simulink library "ChimeSignalGeneratorLibBtc"  (R2022b)
settings: Solver=VariableStepAuto  StartTime=0.0  StopTime=10.0  RelTol=1e-3
libraries: simulink x12, dspmathops x3, FeaturePath x1, HandyTextFile x1, RTC x1
(part 1 of 2)
settings Model: Creator=kl13806  LastModifiedBy=kl13806
settings SolverCC: AlgebraicLoopSolver=TrustRegion
settings DebuggingCC: UnconnectedInputMsg=warning  UnconnectedOutputMsg=warning  UnconnectedLineMsg=warning  SFMachineParentedDataDiag=warning
settings ModelReferenceCC: EnableRefExpFcnMdlSchedulingChecks=on
settings RTWCC: DLArmComputeVersion=19.05

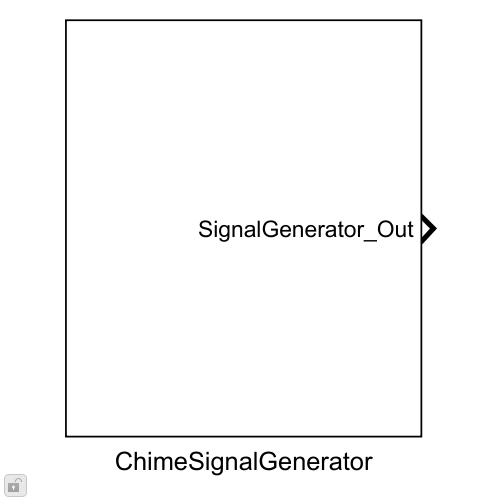
[thumbnail: Simulink's stored preview of the top-level diagram]
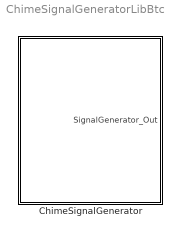
== system ChimeSignalGeneratorLibBtc ==
  ChimeSignalGenerator : Subsystem  mask(Chimes ChimeSignalGenerator){Config=[], FeatureName=SignalGenerator}
      mask prompts: Config "ChimeSignalGeneratorConfig"; FeatureName "Feature path name:"
      mask init:
      | blkh=gcbh;
      | Config=BTConfig.Assert(blkh,Config);
      | 
      | Config.Validate();
      | 
      | BTConfig.InitSetFeatureIfPresent(blkh,'FeatureName');
      | 
      | % Flatten for MFBs
      | frameSize_samples = Config.FrameSizeSamples;
      mask Callback Config: BTConfig.CallbackHideIfPresent(gcbh,{'FeatureName'});
      mask TypeOptions FeatureName: FeaturePath/FeatureName

== system ChimeSignalGeneratorLibBtc/ChimeSignalGenerator ==
  FeaturePath : FeaturePath/FeaturePath  FeatureName=SignalGenerator  IsGroup=off  GroupNumber=-1  IsModule=off  TriggerInit=[345 -266 495 -144]
  For Each Subsystem : Subsystem  TreatAsAtomicUnit=on
  HandyDefaultConfigFile : HandyTextFile/HandyTextFile  TemplateSource=Config  FileSuffix=Init  OpenDialogOnLoad=off  UseThisBlockName=off  TheDefaultText=|  ShowInLibBrowser=on
      | % $(FILENAME) Setup model parameters for each "Init" callback (e.g. update diagram)
      | sample_rate_in_hertz = 44100;
      | frame_size = 32;
      | sysin_channel_count = 2;
  RTC : RTC/RTC  Description=It is LinearSignal generator block  REQ_Priority=RTC_Mask.NormalPriority  RequestAtInit=off  EnableRequest=off  REQElemName1=ChimesMode  REQElemType1=int32  REQElemWidth1=length(Config.SelectMode)  REQElemInitial1=[Config.SelectMode]  REQElemName2=StartingFrequency  REQElemType2=single  REQElemWidth2=length(Config.StartFreqHz)  REQElemInitial2=[Config.StartFreqHz]  REQElemName3=EndingFrequency  REQElemType3=single  REQElemWidth3=length(Config.EndFreqHz)  REQElemInitial3=[Config.EndFreqHz]  REQElemName4=Steps  REQElemType4=single  REQElemWidth4=length(Config.SweepTimeSec)  REQElemInitial4=[Config.SweepTimeSec]  REQElemName5=StartingPhase  REQElemType5=single  REQElemWidth5=length(Config.StartPhaseRad)  REQElemInitial5=[Config.StartPhaseRad]  REQElemName6=ToneGains  REQElemType6=single  REQElemWidth6=length(Config.ToneGains)  REQElemInitial6=[Config.ToneGains]  REQElemName7=RandomNoise  REQElemType7=single  REQElemWidth7=length(Config.RandomNoise)  REQElemInitial7=[Config.RandomNoise]  REQElemName8=CyclesPerSteps  REQElemType8=int32  REQElemWidth8=length(Config.CyclesPerStep)  REQElemInitial8=[Config.CyclesPerStep]  REQElemType9=uint32  REQElemWidth9=1  REQElemInitial9=[]  REQElemType10=uint32  REQElemWidth10=1  REQElemInitial10=[]  EnableResponse=on  EnableRSP_StatusIn=off  RSPElemType1=uint32  RSPElemWidth1=1  RSPElemType2=uint32  RSPElemWidth2=1  RSPElemType3=uint32  RSPElemWidth3=1  RSPElemType4=uint32  RSPElemWidth4=1  RSPElemType5=uint32  RSPElemWidth5=1  RSPElemType6=uint32  RSPElemWidth6=1  RSPElemType7=uint32  RSPElemWidth7=1  RSPElemType8=uint32  RSPElemWidth8=1  RSPElemType9=uint32  RSPElemWidth9=1  RSPElemType10=uint32  RSPElemWidth10=1  EnableNotification=off  EnableNTF_PrepTrig=off  NTFElemType1=uint32  NTFElemWidth1=1  NTFElemType2=uint32  NTFElemWidth2=1  NTFElemType3=uint32  NTFElemWidth3=1  NTFElemType4=uint32  NTFElemWidth4=1  NTFElemType5=uint32  NTFElemWidth5=1  NTFElemType6=uint32  NTFElemWidth6=1  NTFElemType7=uint32  NTFElemWidth7=1  NTFElemType8=uint32  NTFElemWidth8=1  NTFElemType9=uint32  NTFElemWidth9=1  NTFElemType10=uint32  NTFElemWidth10=1  MaskMessageName=Set
  Transpose{,1..7} (8 alike) : Math  Operator=transpose  SignedPower=on
  SignalGenerator_Out : Outport  PortDimensions=[Config.FrameSizeSamples length(Config.SelectMode)]  VectorParamsAs1DForOutWhenUnconnected=off
  wires:
  Transpose7/1 -> For Each Subsystem/7(RandomNoise)  "tone_gains"
  RTC/4 -> Transpose3/1  "steps"
  Transpose6/1 -> For Each Subsystem/8(CyclesPerSteps)  "cycels_per_steps"
  RTC/8 -> Transpose6/1  "cycels_per_steps"
  Transpose5/1 -> For Each Subsystem/2(StartFrequency)  "start_freq"
  Transpose4/1 -> For Each Subsystem/3(EndFrequency)  "end_freq"
  Transpose3/1 -> For Each Subsystem/4(Steps)  "steps"
  Transpose1/1 -> For Each Subsystem/5(StartingPhase)  "start_phase"
  Transpose2/1 -> For Each Subsystem/6(ToneGains)  "tone_gains"
  RTC/7 -> Transpose7/1  "random_noise"
  Transpose/1 -> For Each Subsystem/1(mode)  "chime_mode"
  RTC/1 -> Transpose/1  "chime_mode"
  RTC/6 -> Transpose2/1  "tone_gains"
  RTC/5 -> Transpose1/1  "start_phase"
  RTC/3 -> Transpose4/1  "end_freq"
  RTC/2 -> Transpose5/1  "start_freq"
  For Each Subsystem/1(Out) -> SignalGenerator_Out/1

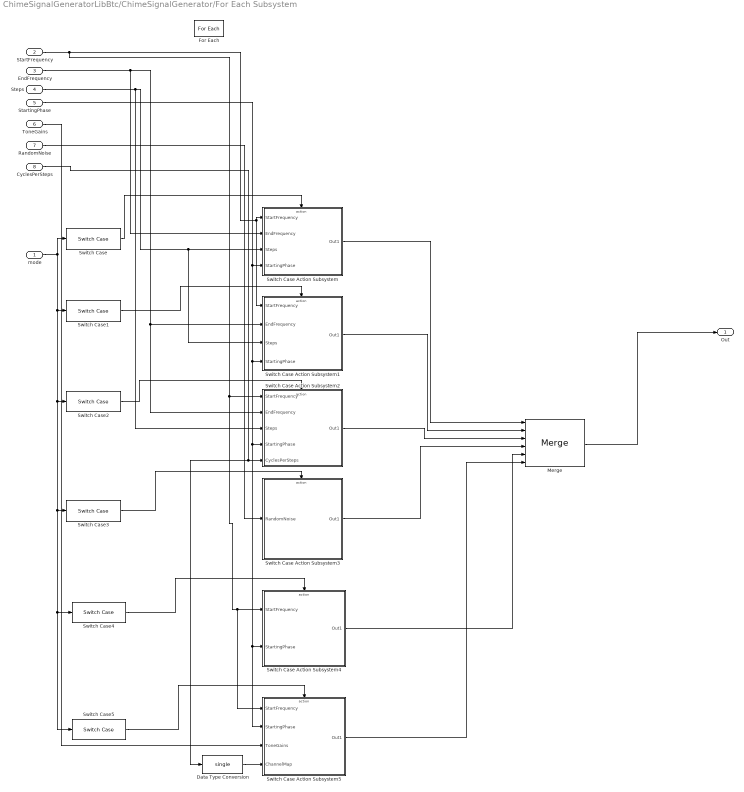
== system ChimeSignalGeneratorLibBtc/ChimeSignalGenerator/For Each Subsystem ==
  mode : Inport  Partition=on  PartitionDimension=2  PartitionWidth=1  PartitionOffset=0
  StartFrequency : Inport  Port=2  Partition=on  PartitionDimension=2  PartitionWidth=2  PartitionOffset=0
  EndFrequency : Inport  Port=3  Partition=on  PartitionDimension=2  PartitionWidth=2  PartitionOffset=0
  Steps : Inport  Port=4  Partition=on  PartitionDimension=2  PartitionWidth=2  PartitionOffset=0
  StartingPhase : Inport  Port=5  Partition=on  PartitionDimension=2  PartitionWidth=2  PartitionOffset=0
  ToneGains : Inport  Port=6  Partition=on  PartitionDimension=2  PartitionWidth=2  PartitionOffset=0
  RandomNoise : Inport  Port=7  Partition=on  PartitionDimension=2  PartitionWidth=2  PartitionOffset=0
  CyclesPerSteps : Inport  Port=8  Partition=on  PartitionDimension=2  PartitionWidth=2  PartitionOffset=0
  Data Type Conversion : DataTypeConversion  OutDataTypeStr=single  SaturateOnIntegerOverflow=off  RndMeth=Floor
  For Each : ForEach  DisableCoverage=on
  Merge : Merge  Inputs=6
  Switch Case : SwitchCase  ShowDefaultCase=off
  Switch Case Action Subsystem : Subsystem  TreatAsAtomicUnit=on
  Switch Case Action Subsystem1 : Subsystem  TreatAsAtomicUnit=on
  Switch Case Action Subsystem2 : Subsystem  TreatAsAtomicUnit=on
  Switch Case Action Subsystem3 : Subsystem  TreatAsAtomicUnit=on
  Switch Case Action Subsystem4 : Subsystem  TreatAsAtomicUnit=on
  Switch Case Action Subsystem5 : Subsystem  TreatAsAtomicUnit=on
  Switch Case1 : SwitchCase  CaseConditions={2}  ShowDefaultCase=off
  Switch Case2 : SwitchCase  CaseConditions={3}  ShowDefaultCase=off
  Switch Case3 : SwitchCase  CaseConditions={4}  ShowDefaultCase=off
  Switch Case4 : SwitchCase  CaseConditions={5}  ShowDefaultCase=off
  Switch Case5 : SwitchCase  CaseConditions={6}  ShowDefaultCase=off
  Out : Outport  ConcatenationDimension=2
  wires:
  StartFrequency/1 -> Switch Case Action Subsystem5/1(StartFrequency), Switch Case Action Subsystem4/1(StartFrequency), Switch Case Action Subsystem2/1(StartFrequency), Switch Case Action Subsystem1/1(StartFrequency), Switch Case Action Subsystem/1(StartFrequency)
  mode/1 -> Switch Case5/1, Switch Case4/1, Switch Case3/1, Switch Case2/1, Switch Case1/1, Switch Case/1
  Switch Case/1 -> Switch Case Action Subsystem/Action
  Switch Case1/1 -> Switch Case Action Subsystem1/Action
  Switch Case2/1 -> Switch Case Action Subsystem2/Action
  Switch Case3/1 -> Switch Case Action Subsystem3/Action
  Switch Case4/1 -> Switch Case Action Subsystem4/Action
  Switch Case5/1 -> Switch Case Action Subsystem5/Action
  Switch Case Action Subsystem3/1(Out1) -> Merge/4
  Switch Case Action Subsystem4/1(Out1) -> Merge/5
  EndFrequency/1 -> Switch Case Action Subsystem/2(EndFrequency), Switch Case Action Subsystem2/2(EndFrequency), Switch Case Action Subsystem1/2(EndFrequency)
  Steps/1 -> Switch Case Action Subsystem1/3(Steps), Switch Case Action Subsystem/3(Steps), Switch Case Action Subsystem2/3(Steps)
  StartingPhase/1 -> Switch Case Action Subsystem/4(StartingPhase), Switch Case Action Subsystem5/2(StartingPhase), Switch Case Action Subsystem4/2(StartingPhase), Switch Case Action Subsystem2/4(StartingPhase), Switch Case Action Subsystem1/4(StartingPhase)
  ToneGains/1 -> Switch Case Action Subsystem5/3(ToneGains)
  RandomNoise/1 -> Switch Case Action Subsystem3/1(RandomNoise)
  CyclesPerSteps/1 -> Data Type Conversion/1, Switch Case Action Subsystem2/5(CyclesPerSteps)
  Switch Case Action Subsystem/1(Out1) -> Merge/1
  Switch Case Action Subsystem1/1(Out1) -> Merge/2
  Switch Case Action Subsystem2/1(Out1) -> Merge/3
  Merge/1 -> Out/1
  Data Type Conversion/1 -> Switch Case Action Subsystem5/4(ChannelMap)
  Switch Case Action Subsystem5/1(Out1) -> Merge/6

== system ChimeSignalGeneratorLibBtc/ChimeSignalGenerator/For Each Subsystem/Switch Case Action Subsystem ==
  StartFrequency : Inport
  EndFrequency : Inport  Port=2
  Steps : Inport  Port=3
  StartingPhase : Inport  Port=4
  Action Port : ActionPort
  Log Sweep Signal Generator : Subsystem
  Out1 : Outport
  wires:
  StartFrequency/1 -> Log Sweep Signal Generator/1(start_freq_Hz)
  EndFrequency/1 -> Log Sweep Signal Generator/2(end_freq_Hz)
  Steps/1 -> Log Sweep Signal Generator/3(sweep_time_sec)
  StartingPhase/1 -> Log Sweep Signal Generator/4(start_phase_rad)
  Log Sweep Signal Generator/1(Log_Sweep_Out) -> Out1/1

== system ChimeSignalGeneratorLibBtc/ChimeSignalGenerator/For Each Subsystem/Switch Case Action Subsystem1 ==
  StartFrequency : Inport
  EndFrequency : Inport  Port=2
  Steps : Inport  Port=3
  StartingPhase : Inport  Port=4
  Action Port : ActionPort
  Linear Sweep Signal Generator : Subsystem
  Out1 : Outport
  wires:
  StartFrequency/1 -> Linear Sweep Signal Generator/1(start_freq_Hz)
  EndFrequency/1 -> Linear Sweep Signal Generator/2(end_freq_Hz)
  Steps/1 -> Linear Sweep Signal Generator/3(sweep_time_sec)
  StartingPhase/1 -> Linear Sweep Signal Generator/4(start_phase_rad)
  Linear Sweep Signal Generator/1(Linear_Sweep_Out) -> Out1/1

== system ChimeSignalGeneratorLibBtc/ChimeSignalGenerator/For Each Subsystem/Switch Case Action Subsystem2 ==
  StartFrequency : Inport
  EndFrequency : Inport  Port=2
  Steps : Inport  Port=3
  StartingPhase : Inport  Port=4
  CyclesPerSteps : Inport  Port=5
  Action Port : ActionPort
  Old Sweep Signal Generator : Subsystem
  Out1 : Outport
  wires:
  StartFrequency/1 -> Old Sweep Signal Generator/1(start_freq_Hz)
  EndFrequency/1 -> Old Sweep Signal Generator/2(end_freq_Hz)
  Steps/1 -> Old Sweep Signal Generator/3(steps)
  StartingPhase/1 -> Old Sweep Signal Generator/4(start_phase_rad)
  CyclesPerSteps/1 -> Old Sweep Signal Generator/5(cycles_per_step)
  Old Sweep Signal Generator/1(Old_sweep_Out) -> Out1/1

== system ChimeSignalGeneratorLibBtc/ChimeSignalGenerator/For Each Subsystem/Switch Case Action Subsystem3 ==
  RandomNoise : Inport
  Action Port : ActionPort
  SigGen_Noise : Subsystem  TreatAsAtomicUnit=on
  Out1 : Outport
  wires:
  RandomNoise/1 -> SigGen_Noise/1(random_noise_input)
  SigGen_Noise/1(Noise_Out) -> Out1/1

== system ChimeSignalGeneratorLibBtc/ChimeSignalGenerator/For Each Subsystem/Switch Case Action Subsystem4 ==
  StartFrequency : Inport
  StartingPhase : Inport  Port=2
  Action Port : ActionPort
  SigGen_Sawtooth : Subsystem  TreatAsAtomicUnit=on
  Out1 : Outport
  wires:
  StartFrequency/1 -> SigGen_Sawtooth/1(StartFreq)
  StartingPhase/1 -> SigGen_Sawtooth/2(start_phase)
  SigGen_Sawtooth/1(Output) -> Out1/1

== system ChimeSignalGeneratorLibBtc/ChimeSignalGenerator/For Each Subsystem/Switch Case Action Subsystem5 ==
  StartFrequency : Inport
  StartingPhase : Inport  Port=2
  ToneGains : Inport  Port=3
  ChannelMap : Inport  Port=4
  Action Port : ActionPort
  SigGen_Multitone : Subsystem
  Out1 : Outport
  wires:
  StartFrequency/1 -> SigGen_Multitone/1(start_freq_Hz)
  SigGen_Multitone/1(Multitone_Out) -> Out1/1  "multitone_output"
  StartingPhase/1 -> SigGen_Multitone/2(start_phase_rad)
  ChannelMap/1 -> SigGen_Multitone/4(ChannelMap)
  ToneGains/1 -> SigGen_Multitone/3(ToneGains)

== system ChimeSignalGeneratorLibBtc/ChimeSignalGenerator/For Each Subsystem/Switch Case Action Subsystem/Log Sweep Signal Generator ==
  start_freq_Hz : Inport
  end_freq_Hz : Inport  Port=2
  sweep_time_sec : Inport  Port=3
  start_phase_rad : Inport  Port=4
  Log Sweep Engine : Subsystem  TreatAsAtomicUnit=on
  Log sweep analysis : Subsystem  Commented=on
  To Workspace : ToWorkspace  Commented=on  VariableName=LogSweepOutput  SampleTime=-1
      settings: Save2DSignal=2-D array (concatenate along first dimension)
  Log_Sweep_Out : Outport  VectorParamsAs1DForOutWhenUnconnected=off
  wires:
  Log Sweep Engine/1(Log_Sweep_Out) -> Log sweep analysis/1(In1), To Workspace/1, Log_Sweep_Out/1
  start_freq_Hz/1 -> Log Sweep Engine/1(start_freq_In)
  end_freq_Hz/1 -> Log Sweep Engine/2(end_freq_In)
  sweep_time_sec/1 -> Log Sweep Engine/3(sweep_time_In)
  start_phase_rad/1 -> Log Sweep Engine/4(start_phase_In)

== system ChimeSignalGeneratorLibBtc/ChimeSignalGenerator/For Each Subsystem/Switch Case Action Subsystem1/Linear Sweep Signal Generator ==
  start_freq_Hz : Inport
  end_freq_Hz : Inport  Port=2
  sweep_time_sec : Inport  Port=3
  start_phase_rad : Inport  Port=4
  Linear Sweep Engine : Subsystem  TreatAsAtomicUnit=on
  Linear sweep analysis : Subsystem  Commented=on
  To Workspace1 : ToWorkspace  Commented=on  VariableName=LinearSweepOutput  SampleTime=-1
      settings: Save2DSignal=2-D array (concatenate along first dimension)
  Linear_Sweep_Out : Outport  VectorParamsAs1DForOutWhenUnconnected=off
  wires:
  start_freq_Hz/1 -> Linear Sweep Engine/1(start_freq_In)
  end_freq_Hz/1 -> Linear Sweep Engine/2(end_freq_In)
  sweep_time_sec/1 -> Linear Sweep Engine/3(sweep_time_In)
  start_phase_rad/1 -> Linear Sweep Engine/4(start_phase_In)
  Linear Sweep Engine/1(Linear_Sweep_Out) -> To Workspace1/1, Linear_Sweep_Out/1, Linear sweep analysis/1(In1)

== system ChimeSignalGeneratorLibBtc/ChimeSignalGenerator/For Each Subsystem/Switch Case Action Subsystem2/Old Sweep Signal Generator ==
  start_freq_Hz : Inport
  end_freq_Hz : Inport  Port=2
  steps : Inport  Port=3
  start_phase_rad : Inport  Port=4
  cycles_per_step : Inport  Port=5
  Old Sweep Engine : Subsystem  TreatAsAtomicUnit=on
  Old sine sweep analysis : Subsystem  Commented=on
  To Workspace5 : ToWorkspace  Commented=on  VariableName=OldSweepOutput  SampleTime=-1
      settings: Save2DSignal=2-D array (concatenate along first dimension)
  Old_sweep_Out : Outport  VectorParamsAs1DForOutWhenUnconnected=off
  wires:
  Old Sweep Engine/1(Old_Sweep_Out) -> To Workspace5/1, Old_sweep_Out/1, Old sine sweep analysis/1(In1)
  start_freq_Hz/1 -> Old Sweep Engine/1(start_freq_In)
  end_freq_Hz/1 -> Old Sweep Engine/2(end_freq_In)
  steps/1 -> Old Sweep Engine/3(steps_In)
  start_phase_rad/1 -> Old Sweep Engine/4(start_phase_In)
  cycles_per_step/1 -> Old Sweep Engine/5(cycles_per_step)

== system ChimeSignalGeneratorLibBtc/ChimeSignalGenerator/For Each Subsystem/Switch Case Action Subsystem3/SigGen_Noise ==
  random_noise_input : Inport
  For Iterator Subsystem : Subsystem  TreatAsAtomicUnit=on
  Noise_Out : Outport  VectorParamsAs1DForOutWhenUnconnected=off
  wires:
  For Iterator Subsystem/1(Out1) -> Noise_Out/1
  random_noise_input/1 -> For Iterator Subsystem/1(InitSeed)  "random_noise"

== system ChimeSignalGeneratorLibBtc/ChimeSignalGenerator/For Each Subsystem/Switch Case Action Subsystem4/SigGen_Sawtooth ==
  StartFreq : Inport
  start_phase : Inport  Port=2
  Add : Sum
  Data Type Conversion : DataTypeConversion  OutDataTypeStr=double  SaturateOnIntegerOverflow=off  RndMeth=Floor
  Data Type Conversion1 : DataTypeConversion  OutDataTypeStr=single  SaturateOnIntegerOverflow=off  RndMeth=Floor
  Divide1 : Product  Inputs=*/
  For Iterator Subsystem : Subsystem  TreatAsAtomicUnit=on
  Mod : Math  Operator=mod  SignedPower=on
  module_phase : Constant  Value=1.0
  sampling_frequency : Constant  Value=Config.FsHz  OutDataTypeStr=single  SampleTime=Inf
  sawtooth_offset : Constant  Value=0.5  OutDataTypeStr=single
  Output : Outport  VectorParamsAs1DForOutWhenUnconnected=off
  wires:
  Mod/1 -> Data Type Conversion1/1  "initial_phase"
  Add/1 -> For Iterator Subsystem/1(IndexStart)  "index_start"
  Data Type Conversion1/1 -> Add/1
  For Iterator Subsystem/1(Out1) -> Output/1
  StartFreq/1 -> Divide1/1
  module_phase/1 -> Mod/2, For Iterator Subsystem/4(ModulePhase)
  sampling_frequency/1 -> Divide1/2
  sawtooth_offset/1 -> For Iterator Subsystem/2(SawtoothOffset), Add/2
  Divide1/1 -> For Iterator Subsystem/3(IncStart)  "inc_start"
  start_phase/1 -> Data Type Conversion/1
  Data Type Conversion/1 -> Mod/1

== system ChimeSignalGeneratorLibBtc/ChimeSignalGenerator/For Each Subsystem/Switch Case Action Subsystem5/SigGen_Multitone ==
  start_freq_Hz : Inport
  start_phase_rad : Inport  Port=2
  ToneGains : Inport  Port=3
  ChannelMap : Inport  Port=4
  Multitone Engine : Subsystem  TreatAsAtomicUnit=on
  Multitone_Out : Outport  VectorParamsAs1DForOutWhenUnconnected=off
  wires:
  ChannelMap/1 -> Multitone Engine/4(ChannelMap)
  Multitone Engine/1(Multitone_Out) -> Multitone_Out/1
  start_phase_rad/1 -> Multitone Engine/2(start_phase_In)  "start_phase"
  start_freq_Hz/1 -> Multitone Engine/1(start_freq_In)  "start_freq"
  ToneGains/1 -> Multitone Engine/3(ToneGains)

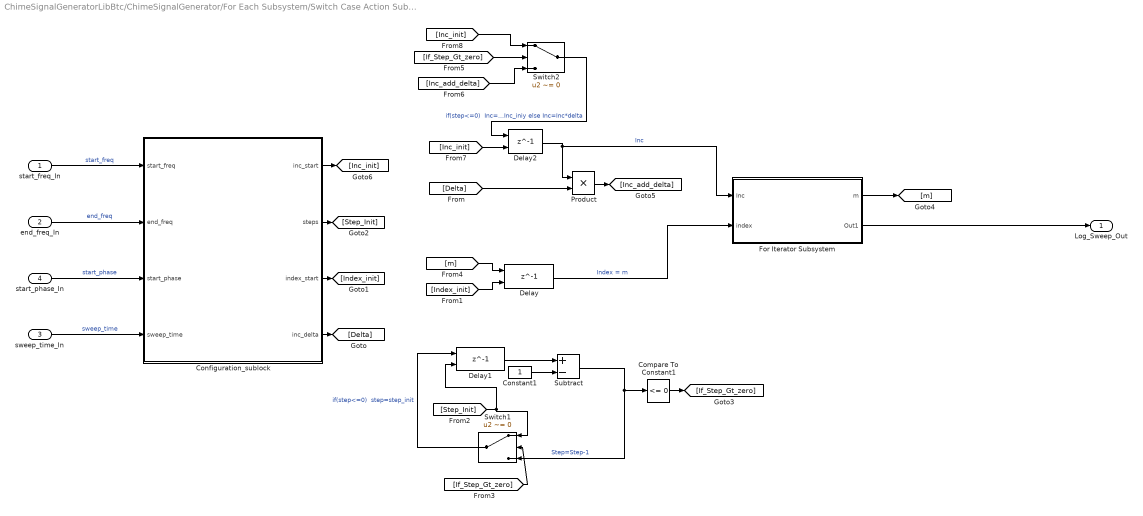
== system ChimeSignalGeneratorLibBtc/ChimeSignalGenerator/For Each Subsystem/Switch Case Action Subsystem/Log Sweep Signal Generator/Log Sweep Engine ==
  start_freq_In : Inport
  end_freq_In : Inport  Port=2
  sweep_time_In : Inport  Port=3
  start_phase_In : Inport  Port=4
  Compare To Constant1 : simulink/Logic and Bit Operations/Compare To Constant  relop=<=  const=0  OutDataTypeStr=boolean
  Configuration_sublock : Subsystem
  Constant1 : Constant  OutDataTypeStr=single
  Delay : Delay  DelayLength=1  InitialConditionSource=Input port
      settings: InputPortMap=u0,p4
  Delay1 : Delay  DelayLength=1  InitialConditionSource=Input port
      settings: InputPortMap=u0,p4
  Delay2 : Delay  DelayLength=1  InitialConditionSource=Input port
      settings: InputPortMap=u0,p4
  For Iterator Subsystem : Subsystem  TreatAsAtomicUnit=on
  Product : Product
  Subtract : Sum  Inputs=+-
  Switch1 : Switch  Criteria=u2 ~= 0  SaturateOnIntegerOverflow=off  InputSameDT=off
  Switch2 : Switch  Criteria=u2 ~= 0  SaturateOnIntegerOverflow=off  InputSameDT=off
  Log_Sweep_Out : Outport  VectorParamsAs1DForOutWhenUnconnected=off
  wires:
  start_freq_In/1 -> Configuration_sublock/1(start_freq)  "start_freq"
  end_freq_In/1 -> Configuration_sublock/2(end_freq)  "end_freq"
  start_phase_In/1 -> Configuration_sublock/3(start_phase)  "start_phase"
  sweep_time_In/1 -> Configuration_sublock/4("sweep_time ")  "sweep_time"
  For Iterator Subsystem/2(Out1) -> Log_Sweep_Out/1
  Configuration_sublock/1(inc_start) -> [Inc_init]
  Configuration_sublock/4(inc_delta) -> [Delta]
  Configuration_sublock/2(steps) -> [Step_Init]
  For Iterator Subsystem/1(m) -> [m]
  Delay/1 -> For Iterator Subsystem/2(index)  "Index = m"
  Subtract/1 -> Switch1/3, Compare To Constant1/1  "Step=Step-1"
  Constant1/1 -> Subtract/2
  Delay1/1 -> Subtract/1
  Switch1/1 -> Delay1/1  "if(step<=0)  step=step_init"
  Delay2/1 -> For Iterator Subsystem/1("Inc "), Product/1  "Inc"
  Configuration_sublock/3(index_start) -> [Index_init]
  [Index_init] -> Delay/2
  [Step_Init] -> Delay1/2, Switch1/1
  Compare To Constant1/1 -> [If_Step_Gt_zero]
  [If_Step_Gt_zero] -> Switch1/2
  [m] -> Delay/1
  [Delta] -> Product/2
  [If_Step_Gt_zero] -> Switch2/2
  Product/1 -> [Inc_add_delta]
  [Inc_add_delta] -> Switch2/3
  [Inc_init] -> Delay2/2
  [Inc_init] -> Switch2/1
  Switch2/1 -> Delay2/1  "if(step<=0)  Inc=Inc_iniy else Inc=Inc*delta"

== system ChimeSignalGeneratorLibBtc/ChimeSignalGenerator/For Each Subsystem/Switch Case Action Subsystem/Log Sweep Signal Generator/Log sweep analysis ==
  In1 : Inport
  Difference : dspmathops/Difference  Run=Yes  dim=Columns  Dimension=1  roundingMode=Floor  overflowMode=off  outputDataTypeStr=Inherit: Same as accumulator  outputMin=[]  outputMax=[]  outputLastDataTypeStr=Inherit: Same as accumulator
  Log Sweep Difference : Scope
  Log Sweep Spectrum Analyzer : SpectrumAnalyzer
  wires:
  Difference/1 -> Log Sweep Difference/1
  In1/1 -> Log Sweep Spectrum Analyzer/1, Difference/1

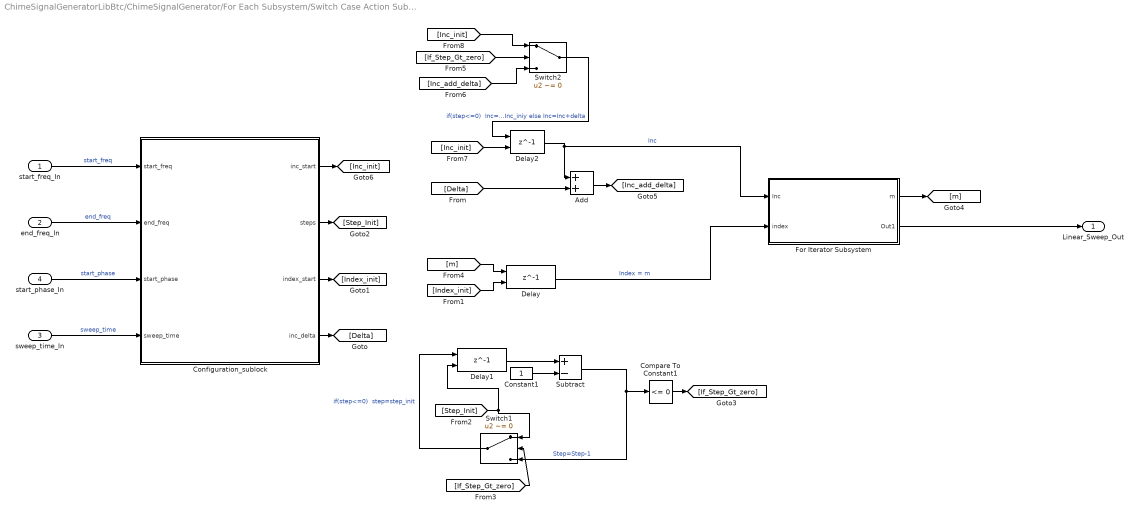
== system ChimeSignalGeneratorLibBtc/ChimeSignalGenerator/For Each Subsystem/Switch Case Action Subsystem1/Linear Sweep Signal Generator/Linear Sweep Engine ==
  start_freq_In : Inport
  end_freq_In : Inport  Port=2
  sweep_time_In : Inport  Port=3
  start_phase_In : Inport  Port=4
  Add : Sum
  Compare To Constant1 : simulink/Logic and Bit Operations/Compare To Constant  relop=<=  const=0  OutDataTypeStr=boolean
  Configuration_sublock : Subsystem
  Constant1 : Constant  OutDataTypeStr=single
  Delay : Delay  DelayLength=1  InitialConditionSource=Input port
      settings: InputPortMap=u0,p4
  Delay1 : Delay  DelayLength=1  InitialConditionSource=Input port
      settings: InputPortMap=u0,p4
  Delay2 : Delay  DelayLength=1  InitialConditionSource=Input port
      settings: InputPortMap=u0,p4
  For Iterator Subsystem : Subsystem  TreatAsAtomicUnit=on
  Subtract : Sum  Inputs=+-
  Switch1 : Switch  Criteria=u2 ~= 0  SaturateOnIntegerOverflow=off  InputSameDT=off
  Switch2 : Switch  Criteria=u2 ~= 0  SaturateOnIntegerOverflow=off  InputSameDT=off
  Linear_Sweep_Out : Outport  VectorParamsAs1DForOutWhenUnconnected=off
  wires:
  Delay2/1 -> For Iterator Subsystem/1("Inc "), Add/1  "Inc"
  Configuration_sublock/4(inc_delta) -> [Delta]
  [Delta] -> Add/2
  [m] -> Delay/1
  Switch1/1 -> Delay1/1  "if(step<=0)  step=step_init"
  [Inc_add_delta] -> Switch2/3
  Delay1/1 -> Subtract/1
  [If_Step_Gt_zero] -> Switch2/2
  [Step_Init] -> Delay1/2, Switch1/1
  start_phase_In/1 -> Configuration_sublock/3(start_phase)  "start_phase"
  Compare To Constant1/1 -> [If_Step_Gt_zero]
  Add/1 -> [Inc_add_delta]
  [Inc_init] -> Delay2/2
  Constant1/1 -> Subtract/2
  Configuration_sublock/1(inc_start) -> [Inc_init]
  [Inc_init] -> Switch2/1
  Switch2/1 -> Delay2/1  "if(step<=0)  Inc=Inc_iniy else Inc=Inc+delta"
  [If_Step_Gt_zero] -> Switch1/2
  Subtract/1 -> Switch1/3, Compare To Constant1/1  "Step=Step-1"
  Delay/1 -> For Iterator Subsystem/2(index)  "Index = m"
  start_freq_In/1 -> Configuration_sublock/1(start_freq)  "start_freq"
  For Iterator Subsystem/1(m) -> [m]
  Configuration_sublock/2(steps) -> [Step_Init]
  [Index_init] -> Delay/2
  For Iterator Subsystem/2(Out1) -> Linear_Sweep_Out/1
  end_freq_In/1 -> Configuration_sublock/2(end_freq)  "end_freq"
  sweep_time_In/1 -> Configuration_sublock/4("sweep_time ")  "sweep_time"
  Configuration_sublock/3(index_start) -> [Index_init]

== system ChimeSignalGeneratorLibBtc/ChimeSignalGenerator/For Each Subsystem/Switch Case Action Subsystem1/Linear Sweep Signal Generator/Linear sweep analysis ==
  In1 : Inport
  Difference : dspmathops/Difference  Run=Yes  dim=Columns  Dimension=1  roundingMode=Floor  overflowMode=off  outputDataTypeStr=Inherit: Same as accumulator  outputMin=[]  outputMax=[]  outputLastDataTypeStr=Inherit: Same as accumulator
  Linear Sweep Difference : Scope
  Linear Sweep Spectrum Analyzer : SpectrumAnalyzer
  wires:
  Difference/1 -> Linear Sweep Difference/1
  In1/1 -> Linear Sweep Spectrum Analyzer/1, Difference/1

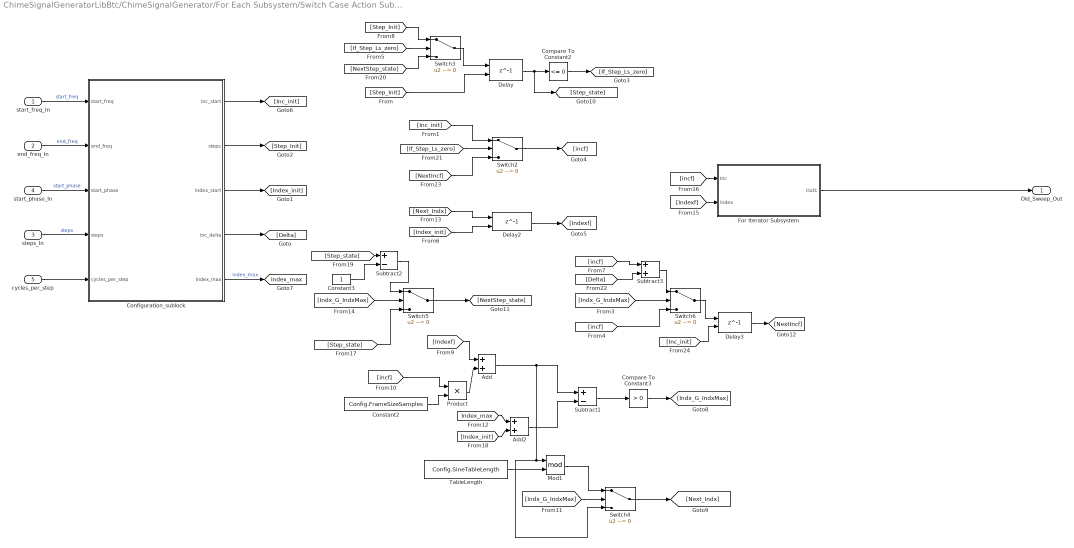
== system ChimeSignalGeneratorLibBtc/ChimeSignalGenerator/For Each Subsystem/Switch Case Action Subsystem2/Old Sweep Signal Generator/Old Sweep Engine ==
  start_freq_In : Inport
  end_freq_In : Inport  Port=2
  steps_In : Inport  Port=3
  start_phase_In : Inport  Port=4
  cycles_per_step : Inport  Port=5
  Add : Sum
  Add2 : Sum  AccumDataTypeStr=single
  Compare To Constant2 : simulink/Logic and Bit Operations/Compare To Constant  relop=<=  const=0  OutDataTypeStr=boolean
  Compare To Constant3 : simulink/Logic and Bit Operations/Compare To Constant  relop=>  const=0  OutDataTypeStr=boolean
  Configuration_sublock : Subsystem
  Constant2 : Constant  Value=Config.FrameSizeSamples  OutDataTypeStr=uint32
  Constant3 : Constant  OutDataTypeStr=single
  Delay : Delay  DelayLength=1  InitialConditionSource=Input port
      settings: InputPortMap=u0,p4
  Delay2 : Delay  DelayLength=1  InitialConditionSource=Input port
      settings: InputPortMap=u0,p4
  Delay3 : Delay  DelayLength=1  InitialConditionSource=Input port
      settings: InputPortMap=u0,p4
  For Iterator Subsystem : Subsystem  TreatAsAtomicUnit=on
  Mod1 : Math  Operator=mod  SignedPower=on
  Product : Product
  Subtract1 : Sum  Inputs=+-
  Subtract2 : Sum  Inputs=+-
  Subtract3 : Sum
  Switch{2..6} (5 alike) : Switch  Criteria=u2 ~= 0  SaturateOnIntegerOverflow=off  InputSameDT=off
  TableLength : Constant  Value=Config.SineTableLength  VectorParams1D=off  OutDataTypeStr=single
  Old_Sweep_Out : Outport  VectorParamsAs1DForOutWhenUnconnected=off
  tag scope: Index_max=global
  wires:
  start_freq_In/1 -> Configuration_sublock/1(start_freq)  "start_freq"
  end_freq_In/1 -> Configuration_sublock/2(end_freq)  "end_freq"
  start_phase_In/1 -> Configuration_sublock/3(start_phase)  "start_phase"
  steps_In/1 -> Configuration_sublock/4("steps ")  "steps"
  For Iterator Subsystem/1(Out1) -> Old_Sweep_Out/1
  Configuration_sublock/1(inc_start) -> [Inc_init]
  Configuration_sublock/4(inc_delta) -> [Delta]
  Configuration_sublock/2(steps) -> [Step_Init]
  Configuration_sublock/3(index_start) -> [Index_init]
  cycles_per_step/1 -> Configuration_sublock/5(cycles_per_step)
  [Indexf] -> For Iterator Subsystem/2(index)
  [incf] -> For Iterator Subsystem/1("Inc ")
  Configuration_sublock/5(index_max) -> [Index_max]  "index_max"
  [Step_Init] -> Delay/2
  Delay/1 -> Compare To Constant2/1, [Step_state]
  Compare To Constant2/1 -> [If_Step_Ls_zero]
  [If_Step_Ls_zero] -> Switch2/2
  [Inc_init] -> Switch2/1
  Switch2/1 -> [incf]
  Delay2/1 -> [Indexf]
  [Index_init] -> Delay2/2
  [If_Step_Ls_zero] -> Switch3/2
  [Step_Init] -> Switch3/1
  Switch3/1 -> Delay/1
  [Indexf] -> Add/1
  [incf] -> Product/1
  Constant2/1 -> Product/2
  Product/1 -> Add/2
  Add/1 -> Switch4/3, Mod1/1, Subtract1/1
  [Index_init] -> Add2/2
  [Index_max] -> Add2/1
  Add2/1 -> Subtract1/2
  Subtract1/1 -> Compare To Constant3/1
  [Indx_G_IndxMax] -> Switch4/2
  TableLength/1 -> Mod1/2
  Mod1/1 -> Switch4/1
  Switch4/1 -> [Next_Indx]
  [Next_Indx] -> Delay2/1
  [Indx_G_IndxMax] -> Switch5/2
  [Step_state] -> Switch5/3
  [Step_state] -> Subtract2/1
  Constant3/1 -> Subtract2/2
  Subtract2/1 -> Switch5/1
  Switch5/1 -> [NextStep_state]
  [NextStep_state] -> Switch3/3
  Compare To Constant3/1 -> [Indx_G_IndxMax]
  [Indx_G_IndxMax] -> Switch6/2
  [incf] -> Switch6/3
  [incf] -> Subtract3/1
  [Delta] -> Subtract3/2
  Subtract3/1 -> Switch6/1
  Switch6/1 -> Delay3/1
  [NextIncf] -> Switch2/3
  [Inc_init] -> Delay3/2
  Delay3/1 -> [NextIncf]

== system ChimeSignalGeneratorLibBtc/ChimeSignalGenerator/For Each Subsystem/Switch Case Action Subsystem2/Old Sweep Signal Generator/Old sine sweep analysis ==
  In1 : Inport
  Difference : dspmathops/Difference  Run=Yes  dim=Columns  Dimension=1  roundingMode=Floor  overflowMode=off  outputDataTypeStr=Inherit: Same as accumulator  outputMin=[]  outputMax=[]  outputLastDataTypeStr=Inherit: Same as accumulator
  Old Sweep Difference : Scope
  Old Sweep Spectrum Analyzer : SpectrumAnalyzer
  wires:
  Difference/1 -> Old Sweep Difference/1
  In1/1 -> Old Sweep Spectrum Analyzer/1, Difference/1

== system ChimeSignalGeneratorLibBtc/ChimeSignalGenerator/For Each Subsystem/Switch Case Action Subsystem3/SigGen_Noise/For Iterator Subsystem ==
  InitSeed : Inport
  Add1 : Sum
  Constant4 : Constant
  Data Type Conversion : DataTypeConversion  OutDataTypeStr=uint32  SaturateOnIntegerOverflow=off  RndMeth=Floor
  Delay1 : Delay  DelayLength=1  InitialConditionSource=Input port
      settings: InputPortMap=u0,p4
  For Iterator : ForIterator  IterationLimit=Config.FrameSizeSamples
  MATLAB Function : MATLAB Function  TreatAsAtomicUnit=on
  Multiply : Product
  Multiply1 : Product
  Subtract : Sum  Inputs=+-
  rnParam1 : Constant  Value=4.656612873077393e-010
  rnParam2 : Constant  Value=1664525
  rnParam3 : Constant  Value=1013904223
  Out1 : Outport  VectorParamsAs1DForOutWhenUnconnected=off
  wires:
  For Iterator/1 -> MATLAB Function/1(Index)
  Data Type Conversion/1 -> Multiply1/1, Multiply/2
  rnParam1/1 -> Multiply/1
  Multiply/1 -> Subtract/1
  rnParam2/1 -> Multiply1/2
  Constant4/1 -> Subtract/2
  Subtract/1 -> MATLAB Function/2(Data)
  Multiply1/1 -> Add1/1
  rnParam3/1 -> Add1/2
  Add1/1 -> Delay1/1
  Delay1/1 -> Data Type Conversion/1
  InitSeed/1 -> Delay1/2
  MATLAB Function/1(y) -> Out1/1

== system ChimeSignalGeneratorLibBtc/ChimeSignalGenerator/For Each Subsystem/Switch Case Action Subsystem4/SigGen_Sawtooth/For Iterator Subsystem ==
  IndexStart : Inport
  SawtoothOffset : Inport  Port=2
  IncStart : Inport  Port=3
  ModulePhase : Inport  Port=4
  Add1 : Sum
  Constant : Constant  Value=-2.0
  Delay : Delay  DelayLength=1  InitialConditionSource=Input port
      settings: InputPortMap=u0,p4
  For Iterator : ForIterator  IterationLimit=Config.FrameSizeSamples
  MATLAB Function : MATLAB Function  TreatAsAtomicUnit=on
  Mod1 : Math  Operator=mod  SignedPower=on
  Multiply : Product
  Subtract : Sum  Inputs=+-
  Out1 : Outport  VectorParamsAs1DForOutWhenUnconnected=off
  wires:
  MATLAB Function/1(y) -> Out1/1
  ModulePhase/1 -> Mod1/2
  SawtoothOffset/1 -> Subtract/2
  IndexStart/1 -> Delay/2  "index_start"
  IncStart/1 -> Add1/2  "inc_start"
  Delay/1 -> Add1/1, Subtract/1  "phase"
  Subtract/1 -> Multiply/1
  Constant/1 -> Multiply/2
  Add1/1 -> Mod1/1
  Mod1/1 -> Delay/1  "initial_phase"
  Multiply/1 -> MATLAB Function/2(Data)
  For Iterator/1 -> MATLAB Function/1(Index)

== system ChimeSignalGeneratorLibBtc/ChimeSignalGenerator/For Each Subsystem/Switch Case Action Subsystem5/SigGen_Multitone/Multitone Engine ==
  start_freq_In : Inport
  start_phase_In : Inport  Port=2
  ToneGains : Inport  Port=3
  ChannelMap : Inport  Port=4
  Add : Sum
  Configuration_sublock : Subsystem
  Delay : Delay  DelayLength=1  InitialConditionSource=Input port
      settings: InputPortMap=u0,p4
  For Iterator Subsystem : Subsystem  TreatAsAtomicUnit=on
  Multitone_Out : Outport  VectorParamsAs1DForOutWhenUnconnected=off
  wires:
  ChannelMap/1 -> For Iterator Subsystem/4(ChannelMap)
  Configuration_sublock/2(index_start) -> [Index_init]  "index_start"
  [Index_init] -> Delay/2
  [m] -> Delay/1
  Delay/1 -> For Iterator Subsystem/2(index)  "m1"
  ToneGains/1 -> For Iterator Subsystem/3(ToneGains)
  [Inc_init] -> Add/1  "inc"
  Add/1 -> For Iterator Subsystem/1("Inc ")
  [Delta] -> Add/2
  For Iterator Subsystem/1(m) -> [m]
  Configuration_sublock/3(inc_delta) -> [Delta]
  Configuration_sublock/1(inc_start) -> [Inc_init]
  For Iterator Subsystem/2(Out1) -> Multitone_Out/1
  start_phase_In/1 -> Configuration_sublock/2(start_phase)  "start_phase"
  start_freq_In/1 -> Configuration_sublock/1(start_freq)  "start_freq"

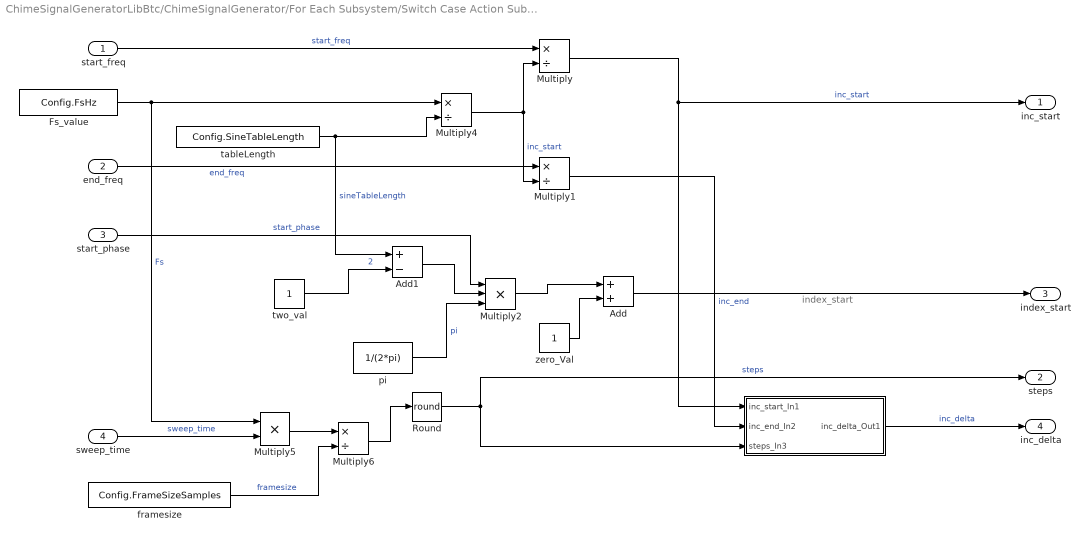
== system ChimeSignalGeneratorLibBtc/ChimeSignalGenerator/For Each Subsystem/Switch Case Action Subsystem/Log Sweep Signal Generator/Log Sweep Engine/Configuration_sublock ==
  note: index_start
  start_freq : Inport
  end_freq : Inport  Port=2
  start_phase : Inport  Port=3
  "sweep_time " : Inport  Port=4
  " " : Subsystem  TreatAsAtomicUnit=on
  Add : Sum
  Add1 : Sum  Inputs=+-
  Fs_value : Constant  Value=Config.FsHz  OutDataTypeStr=single
  Multiply{,1,4,6} (4 alike) : Product  Inputs=*/
  Multiply2 : Product  Inputs=***
  Multiply5 : Product  Inputs=**
  Round : Rounding  Operator=round
  framesize : Constant  Value=Config.FrameSizeSamples  VectorParams1D=off  OutDataTypeStr=uint32
  pi : Constant  Value=1/(2*pi)  VectorParams1D=off  OutDataTypeStr=single
  tableLength : Constant  Value=Config.SineTableLength  VectorParams1D=off  OutDataTypeStr=single
  two_val : Constant  VectorParams1D=off  OutDataTypeStr=uint32
  zero_Val : Constant  VectorParams1D=off  OutDataTypeStr=single
  inc_start : Outport  VectorParamsAs1DForOutWhenUnconnected=off
  steps : Outport  Port=2  VectorParamsAs1DForOutWhenUnconnected=off
  index_start : Outport  Port=3  VectorParamsAs1DForOutWhenUnconnected=off
  inc_delta : Outport  Port=4  VectorParamsAs1DForOutWhenUnconnected=off
  wires:
  start_phase/1 -> Multiply2/1  "start_phase"
  tableLength/1 -> Multiply4/2, Add1/1  "sineTableLength"
  two_val/1 -> Add1/2  "2"
  pi/1 -> Multiply2/3  "pi"
  Add1/1 -> Multiply2/2
  zero_Val/1 -> Add/2
  Fs_value/1 -> Multiply5/1, Multiply4/1  "Fs"
  Multiply2/1 -> Add/1
  start_freq/1 -> Multiply/1  "start_freq"
  end_freq/1 -> Multiply1/1  "end_freq"
  Add/1 -> index_start/1
  Multiply/1 -> " "/1(inc_start_In1), inc_start/1  "inc_start"
  Multiply4/1 -> Multiply1/2, Multiply/2  "inc_start"
  Multiply1/1 -> " "/2(inc_end_In2)  "inc_end"
  "sweep_time "/1 -> Multiply5/2  "sweep_time"
  Multiply5/1 -> Multiply6/1
  framesize/1 -> Multiply6/2  "framesize"
  Multiply6/1 -> Round/1
  Round/1 -> " "/3(steps_In3), steps/1  "steps"
  " "/1(inc_delta_Out1) -> inc_delta/1  "inc_delta"

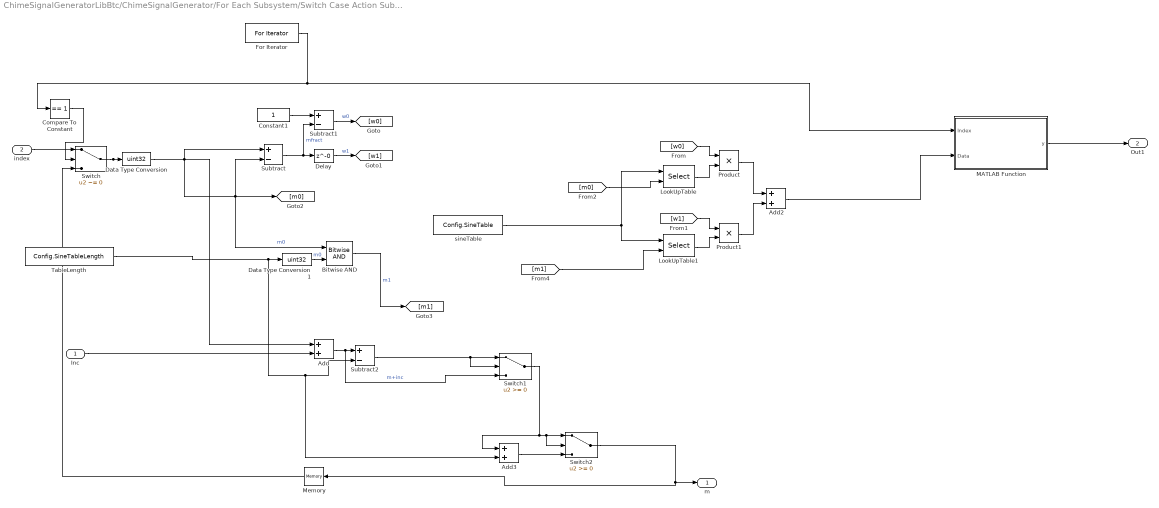
== system ChimeSignalGeneratorLibBtc/ChimeSignalGenerator/For Each Subsystem/Switch Case Action Subsystem/Log Sweep Signal Generator/Log Sweep Engine/For Iterator Subsystem ==
  "Inc " : Inport
  index : Inport  Port=2
  Add : Sum
  Add2 : Sum
  Add3 : Sum
  Bitwise AND : simulink/Logic and Bit Operations/Bitwise Operator  logicop=AND  UseBitMask=off  NumInputPorts=2  BitMask=bin2dec('11011001')  BitMaskRealWorld=Stored Integer
  Compare To Constant : simulink/Logic and Bit Operations/Compare To Constant  relop===  const=1  OutDataTypeStr=boolean
  Constant1 : Constant  OutDataTypeStr=single
  Data Type Conversion : DataTypeConversion  OutDataTypeStr=uint32  SaturateOnIntegerOverflow=off  RndMeth=Floor
  Data Type Conversion1 : DataTypeConversion  OutDataTypeStr=uint32  SaturateOnIntegerOverflow=off  RndMeth=Floor
  Delay : Delay  DelayLength=0
  For Iterator : ForIterator  ResetStates=reset  IterationLimit=Config.FrameSizeSamples
  LookUpTable : Selector  IndexMode=Zero-based  InputPortWidth=Config.SineTableLength  IndexOptions=Index vector (port)  Indices=[1 3]  OutputSizes=1
  LookUpTable1 : Selector  IndexMode=Zero-based  InputPortWidth=Config.SineTableLength  IndexOptions=Index vector (port)  Indices=[1 3]  OutputSizes=1
  MATLAB Function : MATLAB Function  TreatAsAtomicUnit=on
  Memory : Memory  InheritSampleTime=on
  Product : Product
  Product1 : Product
  Subtract : Sum  Inputs=+-  OutDataTypeStr=single
  Subtract1 : Sum  Inputs=+-  OutDataTypeStr=single
  Subtract2 : Sum  Inputs=+-
  Switch : Switch  Criteria=u2 ~= 0  SaturateOnIntegerOverflow=off  InputSameDT=off
  Switch1 : Switch  SaturateOnIntegerOverflow=off  InputSameDT=off
  Switch2 : Switch  SaturateOnIntegerOverflow=off  InputSameDT=off
  TableLength : Constant  Value=Config.SineTableLength  VectorParams1D=off  OutDataTypeStr=single
  sineTable : Constant  Value=Config.SineTable  OutDataTypeStr=single
  m : Outport  VectorParamsAs1DForOutWhenUnconnected=off
  Out1 : Outport  Port=2  VectorParamsAs1DForOutWhenUnconnected=off
  wires:
  Add2/1 -> MATLAB Function/2(Data)
  TableLength/1 -> Data Type Conversion1/1, Add3/2, Subtract2/2
  Compare To Constant/1 -> Switch/2
  index/1 -> Switch/1
  Switch/1 -> Add/1, Data Type Conversion/1
  Add/1 -> Switch1/3, Subtract2/1  "m+inc"
  For Iterator/1 -> MATLAB Function/1(Index), Compare To Constant/1
  Memory/1 -> Switch/3
  Data Type Conversion/1 -> Bitwise AND/1, Subtract/2, [m0], Subtract/1  "m0"
  Subtract/1 -> Delay/1, Subtract1/2  "mfract"
  Constant1/1 -> Subtract1/1
  Subtract1/1 -> [w0]  "w0"
  Delay/1 -> [w1]  "w1"
  sineTable/1 -> LookUpTable1/1, LookUpTable/1
  [m0] -> LookUpTable/2
  [w0] -> Product/1
  LookUpTable/1 -> Product/2
  [m1] -> LookUpTable1/2
  [w1] -> Product1/1
  LookUpTable1/1 -> Product1/2
  Product/1 -> Add2/1
  Product1/1 -> Add2/2
  MATLAB Function/1(y) -> Out1/1
  "Inc "/1 -> Add/2
  Data Type Conversion1/1 -> Bitwise AND/2  "m0"
  Switch1/1 -> Add3/1, Switch2/2, Switch2/1
  Switch2/1 -> Memory/1, m/1
  Subtract2/1 -> Switch1/1, Switch1/2
  Add3/1 -> Switch2/3
  Bitwise AND/1 -> [m1]  "m1"

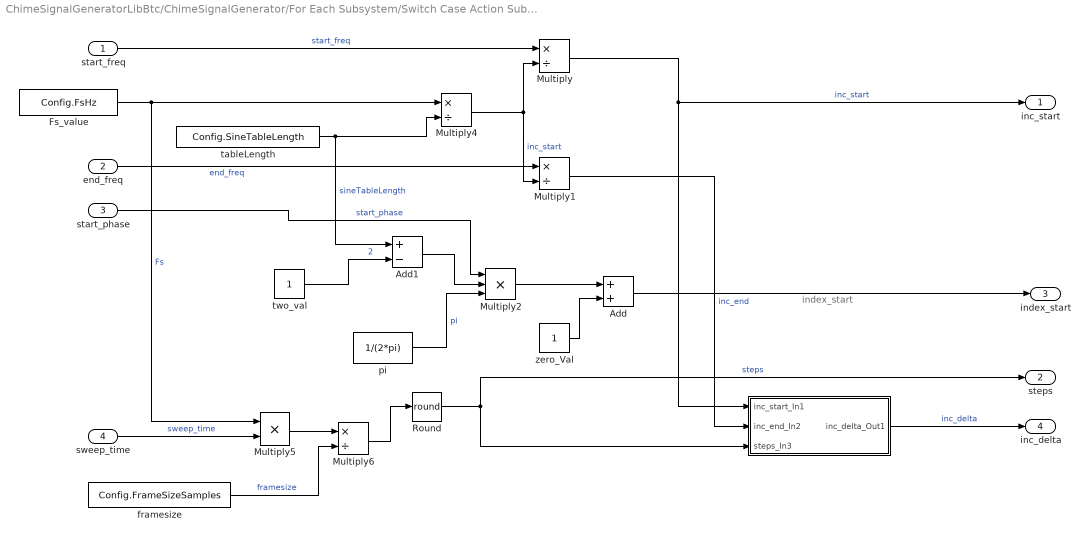
== system ChimeSignalGeneratorLibBtc/ChimeSignalGenerator/For Each Subsystem/Switch Case Action Subsystem1/Linear Sweep Signal Generator/Linear Sweep Engine/Configuration_sublock ==
  note: index_start
  start_freq : Inport
  end_freq : Inport  Port=2
  start_phase : Inport  Port=3
  "sweep_time " : Inport  Port=4
  " " : Subsystem  TreatAsAtomicUnit=on
  Add : Sum
  Add1 : Sum  Inputs=+-
  Fs_value : Constant  Value=Config.FsHz  OutDataTypeStr=single
  Multiply{,1,4,6} (4 alike) : Product  Inputs=*/
  Multiply2 : Product  Inputs=***
  Multiply5 : Product  Inputs=**
  Round : Rounding  Operator=round
  framesize : Constant  Value=Config.FrameSizeSamples  VectorParams1D=off  OutDataTypeStr=uint32
  pi : Constant  Value=1/(2*pi)  VectorParams1D=off  OutDataTypeStr=single
  tableLength : Constant  Value=Config.SineTableLength  VectorParams1D=off  OutDataTypeStr=single
  two_val : Constant  VectorParams1D=off  OutDataTypeStr=uint32
  zero_Val : Constant  VectorParams1D=off  OutDataTypeStr=single
  inc_start : Outport  VectorParamsAs1DForOutWhenUnconnected=off
  steps : Outport  Port=2  VectorParamsAs1DForOutWhenUnconnected=off
  index_start : Outport  Port=3  VectorParamsAs1DForOutWhenUnconnected=off
  inc_delta : Outport  Port=4  VectorParamsAs1DForOutWhenUnconnected=off
  wires:
  Add1/1 -> Multiply2/2
  zero_Val/1 -> Add/2
  two_val/1 -> Add1/2  "2"
  pi/1 -> Multiply2/3  "pi"
  Fs_value/1 -> Multiply5/1, Multiply4/1  "Fs"
  Multiply2/1 -> Add/1
  tableLength/1 -> Multiply4/2, Add1/1  "sineTableLength"
  start_freq/1 -> Multiply/1  "start_freq"
  start_phase/1 -> Multiply2/1  "start_phase"
  end_freq/1 -> Multiply1/1  "end_freq"
  Add/1 -> index_start/1
  Multiply/1 -> " "/1(inc_start_In1), inc_start/1  "inc_start"
  Multiply4/1 -> Multiply1/2, Multiply/2  "inc_start"
  Multiply1/1 -> " "/2(inc_end_In2)  "inc_end"
  "sweep_time "/1 -> Multiply5/2  "sweep_time"
  Multiply5/1 -> Multiply6/1
  framesize/1 -> Multiply6/2  "framesize"
  Multiply6/1 -> Round/1
  Round/1 -> " "/3(steps_In3), steps/1  "steps"
  " "/1(inc_delta_Out1) -> inc_delta/1  "inc_delta"

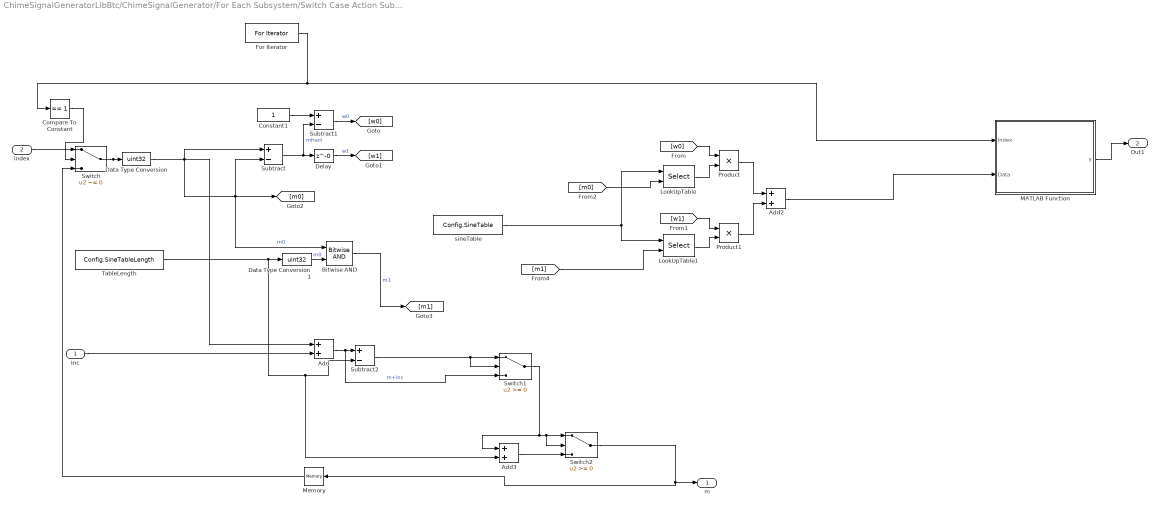
== system ChimeSignalGeneratorLibBtc/ChimeSignalGenerator/For Each Subsystem/Switch Case Action Subsystem1/Linear Sweep Signal Generator/Linear Sweep Engine/For Iterator Subsystem ==
  "Inc " : Inport
  index : Inport  Port=2
  Add : Sum
  Add2 : Sum
  Add3 : Sum
  Bitwise AND : simulink/Logic and Bit Operations/Bitwise Operator  logicop=AND  UseBitMask=off  NumInputPorts=2  BitMask=bin2dec('11011001')  BitMaskRealWorld=Stored Integer
  Compare To Constant : simulink/Logic and Bit Operations/Compare To Constant  relop===  const=1  OutDataTypeStr=boolean
  Constant1 : Constant  OutDataTypeStr=single
  Data Type Conversion : DataTypeConversion  OutDataTypeStr=uint32  SaturateOnIntegerOverflow=off  RndMeth=Floor
  Data Type Conversion1 : DataTypeConversion  OutDataTypeStr=uint32  SaturateOnIntegerOverflow=off  RndMeth=Floor
  Delay : Delay  DelayLength=0
  For Iterator : ForIterator  ResetStates=reset  IterationLimit=Config.FrameSizeSamples
  LookUpTable : Selector  IndexMode=Zero-based  InputPortWidth=Config.SineTableLength  IndexOptions=Index vector (port)  Indices=[1 3]  OutputSizes=1
  LookUpTable1 : Selector  IndexMode=Zero-based  InputPortWidth=Config.SineTableLength  IndexOptions=Index vector (port)  Indices=[1 3]  OutputSizes=1
  MATLAB Function : MATLAB Function  TreatAsAtomicUnit=on
  Memory : Memory  InheritSampleTime=on
  Product : Product
  Product1 : Product
  Subtract : Sum  Inputs=+-  OutDataTypeStr=single
  Subtract1 : Sum  Inputs=+-  OutDataTypeStr=single
  Subtract2 : Sum  Inputs=+-
  Switch : Switch  Criteria=u2 ~= 0  SaturateOnIntegerOverflow=off  InputSameDT=off
  Switch1 : Switch  SaturateOnIntegerOverflow=off  InputSameDT=off
  Switch2 : Switch  SaturateOnIntegerOverflow=off  InputSameDT=off
  TableLength : Constant  Value=Config.SineTableLength  VectorParams1D=off  OutDataTypeStr=single
  sineTable : Constant  Value=Config.SineTable  OutDataTypeStr=single
  m : Outport  VectorParamsAs1DForOutWhenUnconnected=off
  Out1 : Outport  Port=2  VectorParamsAs1DForOutWhenUnconnected=off
  wires:
  Add2/1 -> MATLAB Function/2(Data)
  TableLength/1 -> Data Type Conversion1/1, Add3/2, Subtract2/2
  Compare To Constant/1 -> Switch/2
  index/1 -> Switch/1
  Switch/1 -> Add/1, Data Type Conversion/1
  Add/1 -> Switch1/3, Subtract2/1  "m+inc"
  For Iterator/1 -> MATLAB Function/1(Index), Compare To Constant/1
  Memory/1 -> Switch/3
  Data Type Conversion/1 -> Bitwise AND/1, Subtract/2, [m0], Subtract/1  "m0"
  Subtract/1 -> Delay/1, Subtract1/2  "mfract"
  Constant1/1 -> Subtract1/1
  Subtract1/1 -> [w0]  "w0"
  Delay/1 -> [w1]  "w1"
  sineTable/1 -> LookUpTable1/1, LookUpTable/1
  [m0] -> LookUpTable/2
  [w0] -> Product/1
  LookUpTable/1 -> Product/2
  [m1] -> LookUpTable1/2
  [w1] -> Product1/1
  LookUpTable1/1 -> Product1/2
  Product/1 -> Add2/1
  Product1/1 -> Add2/2
  MATLAB Function/1(y) -> Out1/1
  "Inc "/1 -> Add/2
  Data Type Conversion1/1 -> Bitwise AND/2  "m0"
  Switch1/1 -> Add3/1, Switch2/2, Switch2/1
  Switch2/1 -> Memory/1, m/1
  Subtract2/1 -> Switch1/1, Switch1/2
  Add3/1 -> Switch2/3
  Bitwise AND/1 -> [m1]  "m1"

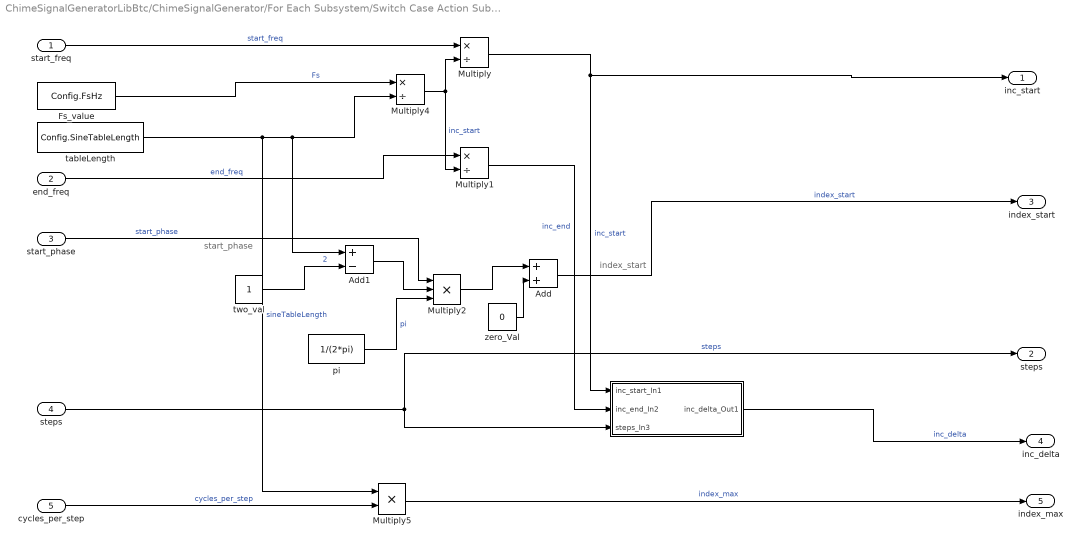
== system ChimeSignalGeneratorLibBtc/ChimeSignalGenerator/For Each Subsystem/Switch Case Action Subsystem2/Old Sweep Signal Generator/Old Sweep Engine/Configuration_sublock ==
  note: index_start
  note: start_phase
  start_freq : Inport
  end_freq : Inport  Port=2
  start_phase : Inport  Port=3
  "steps " : Inport  Port=4
  cycles_per_step : Inport  Port=5
  " " : Subsystem  TreatAsAtomicUnit=on
  Add : Sum
  Add1 : Sum  Inputs=+-
  Fs_value : Constant  Value=Config.FsHz  OutDataTypeStr=single
  Multiply : Product  Inputs=*/
  Multiply1 : Product  Inputs=*/
  Multiply2 : Product  Inputs=***
  Multiply4 : Product  Inputs=*/
  Multiply5 : Product  Inputs=**
  pi : Constant  Value=1/(2*pi)  VectorParams1D=off  OutDataTypeStr=single
  tableLength : Constant  Value=Config.SineTableLength  OutDataTypeStr=single
  two_val : Constant  VectorParams1D=off  OutDataTypeStr=uint32
  zero_Val : Constant  Value=0  OutDataTypeStr=uint32
  inc_start : Outport  VectorParamsAs1DForOutWhenUnconnected=off
  steps : Outport  Port=2  VectorParamsAs1DForOutWhenUnconnected=off
  index_start : Outport  Port=3  VectorParamsAs1DForOutWhenUnconnected=off
  inc_delta : Outport  Port=4  VectorParamsAs1DForOutWhenUnconnected=off
  index_max : Outport  Port=5  VectorParamsAs1DForOutWhenUnconnected=off
  wires:
  start_phase/1 -> Multiply2/1  "start_phase"
  tableLength/1 -> Multiply5/1, Multiply4/2, Add1/1  "sineTableLength"
  two_val/1 -> Add1/2  "2"
  pi/1 -> Multiply2/3  "pi"
  Add1/1 -> Multiply2/2
  Add/1 -> index_start/1  "index_start"
  cycles_per_step/1 -> Multiply5/2  "cycles_per_step"
  Multiply5/1 -> index_max/1  "index_max"
  " "/1(inc_delta_Out1) -> inc_delta/1  "inc_delta"
  "steps "/1 -> " "/3(steps_In3), steps/1  "steps"
  Multiply1/1 -> " "/2(inc_end_In2)  "inc_end"
  Multiply4/1 -> Multiply/2, Multiply1/2  "inc_start"
  Multiply/1 -> inc_start/1, " "/1(inc_start_In1)  "inc_start"
  end_freq/1 -> Multiply1/1  "end_freq"
  start_freq/1 -> Multiply/1  "start_freq"
  Multiply2/1 -> Add/1
  Fs_value/1 -> Multiply4/1  "Fs"
  zero_Val/1 -> Add/2

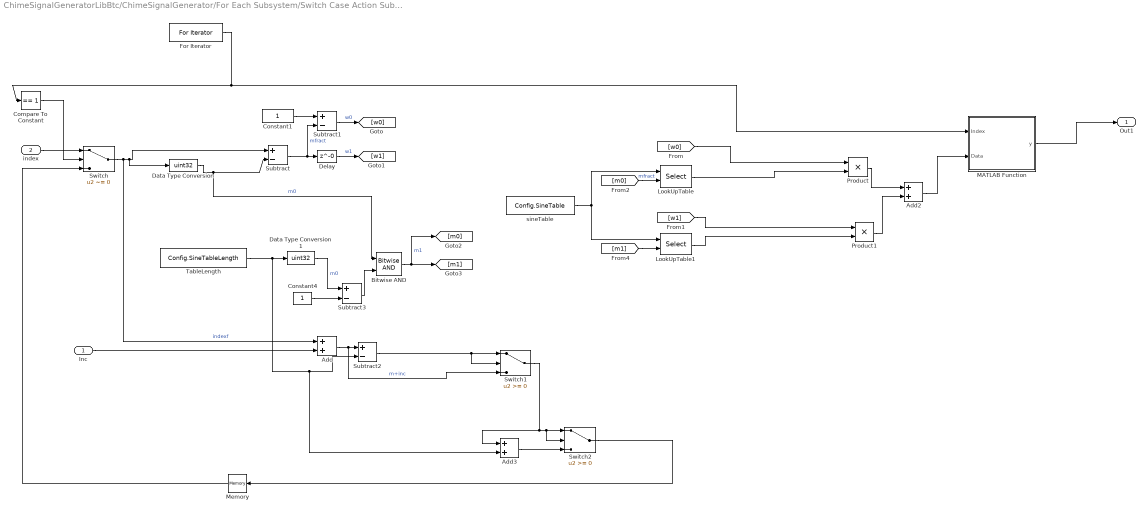
== system ChimeSignalGeneratorLibBtc/ChimeSignalGenerator/For Each Subsystem/Switch Case Action Subsystem2/Old Sweep Signal Generator/Old Sweep Engine/For Iterator Subsystem ==
  "Inc " : Inport
  index : Inport  Port=2
  Add : Sum
  Add2 : Sum
  Add3 : Sum
  Bitwise AND : simulink/Logic and Bit Operations/Bitwise Operator  logicop=AND  UseBitMask=off  NumInputPorts=2  BitMask=bin2dec('11011001')  BitMaskRealWorld=Stored Integer
  Compare To Constant : simulink/Logic and Bit Operations/Compare To Constant  relop===  const=1  OutDataTypeStr=boolean
  Constant1 : Constant  OutDataTypeStr=single
  Constant4 : Constant  OutDataTypeStr=uint32
  Data Type Conversion : DataTypeConversion  OutDataTypeStr=uint32  SaturateOnIntegerOverflow=off  RndMeth=Floor
  Data Type Conversion1 : DataTypeConversion  OutDataTypeStr=uint32  SaturateOnIntegerOverflow=off  RndMeth=Floor
  Delay : Delay  DelayLength=0
  For Iterator : ForIterator  ResetStates=reset  IterationLimit=Config.FrameSizeSamples
  LookUpTable : Selector  IndexMode=Zero-based  InputPortWidth=Config.SineTableLength  IndexOptions=Index vector (port)  Indices=[1 3]  OutputSizes=1
  LookUpTable1 : Selector  IndexMode=Zero-based  InputPortWidth=Config.SineTableLength  IndexOptions=Index vector (port)  Indices=[1 3]  OutputSizes=1
  MATLAB Function : MATLAB Function  TreatAsAtomicUnit=on
  Memory : Memory  InheritSampleTime=on
  Product : Product
  Product1 : Product
  Subtract : Sum  Inputs=+-  OutDataTypeStr=single
  Subtract1 : Sum  Inputs=+-  OutDataTypeStr=single
  Subtract2 : Sum  Inputs=+-
  Subtract3 : Sum  Inputs=+-
  Switch : Switch  Criteria=u2 ~= 0  SaturateOnIntegerOverflow=off  InputSameDT=off
  Switch1 : Switch  SaturateOnIntegerOverflow=off  InputSameDT=off
  Switch2 : Switch  SaturateOnIntegerOverflow=off  InputSameDT=off
  TableLength : Constant  Value=Config.SineTableLength  VectorParams1D=off  OutDataTypeStr=single
  sineTable : Constant  Value=Config.SineTable  OutDataTypeStr=single
  Out1 : Outport  VectorParamsAs1DForOutWhenUnconnected=off
  wires:
  Bitwise AND/1 -> [m0], [m1]  "m1"
  Add3/1 -> Switch2/3
  Subtract2/1 -> Switch1/2, Switch1/1
  Switch2/1 -> Memory/1
  Switch1/1 -> Switch2/1, Switch2/2, Add3/1
  "Inc "/1 -> Add/2
  MATLAB Function/1(y) -> Out1/1
  Product1/1 -> Add2/2
  Product/1 -> Add2/1
  LookUpTable1/1 -> Product1/2
  [w1] -> Product1/1
  [m1] -> LookUpTable1/2
  LookUpTable/1 -> Product/2
  [w0] -> Product/1
  sineTable/1 -> LookUpTable1/1, LookUpTable/1
  Delay/1 -> [w1]  "w1"
  Subtract1/1 -> [w0]  "w0"
  Constant1/1 -> Subtract1/1
  Subtract/1 -> Subtract1/2, Delay/1  "mfract"
  Data Type Conversion/1 -> Subtract/2, Bitwise AND/1  "m0"
  Memory/1 -> Switch/3
  For Iterator/1 -> MATLAB Function/1(Index), Compare To Constant/1
  Add/1 -> Subtract2/1, Switch1/3  "m+inc"
  Switch/1 -> Data Type Conversion/1, Subtract/1, Add/1  "indexf"
  index/1 -> Switch/1
  Compare To Constant/1 -> Switch/2
  TableLength/1 -> Subtract2/2, Add3/2, Data Type Conversion1/1
  Add2/1 -> MATLAB Function/2(Data)
  Data Type Conversion1/1 -> Subtract3/1  "m0"
  Subtract3/1 -> Bitwise AND/2
  Constant4/1 -> Subtract3/2
  [m0] -> LookUpTable/2  "mfract"

== system ChimeSignalGeneratorLibBtc/ChimeSignalGenerator/For Each Subsystem/Switch Case Action Subsystem5/SigGen_Multitone/Multitone Engine/Configuration_sublock ==
  note: index_start
  start_freq : Inport
  start_phase : Inport  Port=2
  Add : Sum
  Fs_value : Constant  Value=Config.FsHz  OutDataTypeStr=single
  Incdelta : Constant  Value=0  OutDataTypeStr=uint32
  Multiply : Product  Inputs=*/
  Multiply1 : Product  Inputs=***
  Multiply4 : Product  Inputs=*/
  Subtract : Sum  Inputs=+-
  constant2 : Constant  OutDataTypeStr=uint32
  tableLength : Constant  Value=Config.SineTableLength  OutDataTypeStr=single
  two_val : Constant  Value=1/(2*pi)  OutDataTypeStr=single
  inc_start : Outport  VectorParamsAs1DForOutWhenUnconnected=off
  index_start : Outport  Port=2  VectorParamsAs1DForOutWhenUnconnected=off
  inc_delta : Outport  Port=3  VectorParamsAs1DForOutWhenUnconnected=off
  wires:
  Incdelta/1 -> inc_delta/1  "inc_delta"
  Multiply4/1 -> Multiply/2
  Multiply/1 -> inc_start/1  "inc_start"
  Add/1 -> index_start/1
  start_phase/1 -> Multiply1/1  "start_phase"
  start_freq/1 -> Multiply/1  "start_freq"
  Multiply1/1 -> Add/1
  tableLength/1 -> Subtract/1, Multiply4/2  "sineTableLength"
  Fs_value/1 -> Multiply4/1  "Fs"
  two_val/1 -> Multiply1/3  "2"
  constant2/1 -> Add/2, Subtract/2
  Subtract/1 -> Multiply1/2
